simulink model "DSO4kW"  (R2024a)
settings: Solver=ode23tb  StartTime=0.0  StopTime=1  MaxStep=1e-5  RelTol=1e-6  AbsTol=1e-6
libraries: spsDiodeLib x10, spsPVArrayLib x9, spsSeriesRLCBranchLib x4, spsCurrentMeasurementLib x2, spsFirstOrderFilterLib x2, spsVoltageMeasurementLib x2, spsIGBTDiodeLib x1, spsPWMGeneratorDCDCLib x1, sps_lib x1
settings Model: Creator=Rahuldev  LastModifiedBy=Rahuldev

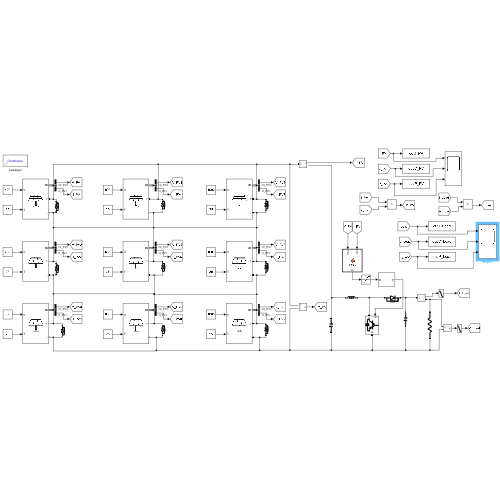
[thumbnail: Simulink's stored preview of the top-level diagram]
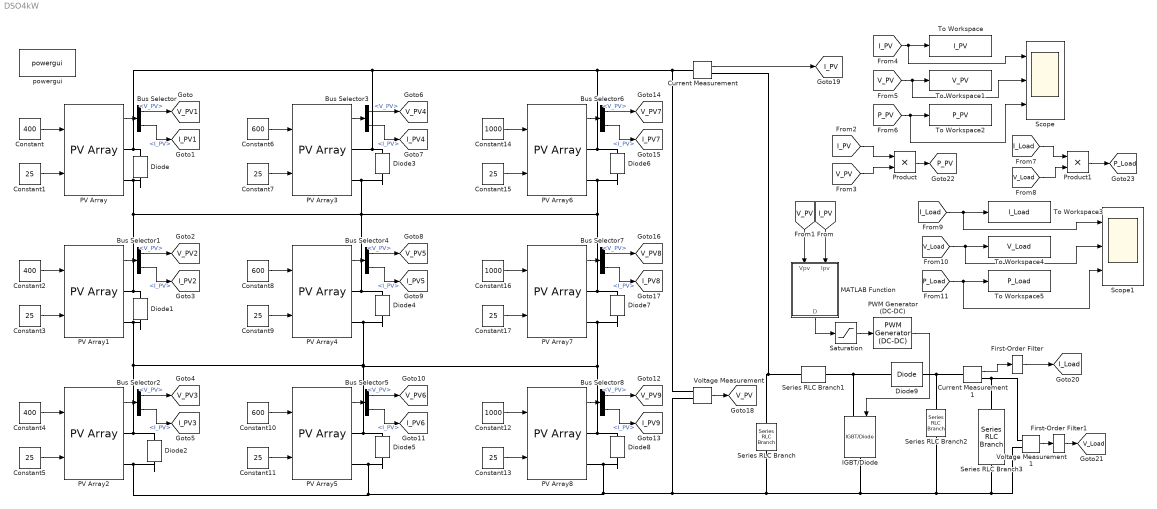
== system DSO4kW ==
  Bus Selector{,1..8} (9 alike) : BusSelector  OutputSignals=V_PV,I_PV
  Constant : Constant  Value=400
  Constant{1,3,5,7,9,11,13,15,17} (9 alike) : Constant  Value=25
  Constant10 : Constant  Value=600
  Constant12 : Constant  Value=1000
  Constant14 : Constant  Value=1000
  Constant16 : Constant  Value=1000
  Constant2 : Constant  Value=400
  Constant4 : Constant  Value=400
  Constant6 : Constant  Value=600
  Constant8 : Constant  Value=600
  Current Measurement : spsCurrentMeasurementLib/Current Measurement  PhasorSimulation=off  OutputType=Complex  PSBequivalent=0
  Current Measurement1 : spsCurrentMeasurementLib/Current Measurement  PhasorSimulation=off  OutputType=Complex  PSBequivalent=0
  Diode{,1..9} (10 alike) : spsDiodeLib/Diode  Ron=0.001  Lon=0  Vf=0.8  IC=0  UseSnubber=0  Rs=500  Cs=250e-9  Measurements=off
  First-Order Filter : spsFirstOrderFilterLib/First-Order Filter  FilterType=Lowpass  Tc=10e-3  Ts=0  Initialize=off  Vac_Init=[0, 0, 60]  Vdc_Init=0  PlotResponse=off  FreqRange="[0,  200,  1]"
  First-Order Filter1 : spsFirstOrderFilterLib/First-Order Filter  FilterType=Lowpass  Tc=10e-3  Ts=0  Initialize=off  Vac_Init=[0, 0, 60]  Vdc_Init=0  PlotResponse=off  FreqRange="[0,  200,  1]"
  IGBT/Diode : spsIGBTDiodeLib/IGBT//Diode  Ron=1e-3  Rs=1e5  Cs=inf  Measurements=off
  MATLAB Function : MATLAB Function  TreatAsAtomicUnit=on
  PV Array{,1..8} (9 alike) : spsPVArrayLib/PV Array  Npar=1  Nser=1  PlotType=array @ 25 deg.C & specified irradiances  S_vec="[ 1000  800  600  400  200 ]"  Temp_C_vec="[ 45 25  ]"  ModuleName=User-defined  PlotWhenSelected=off  Pm=540.474  Ncell=144  Voc=49.32  Isc=13.71  Vm=41.80  Im=12.93  beta_Voc_pc=-0.28  alpha_Isc_pc=0.048  beta_Voc=-0.1381  alpha_Isc=0.0065808  IL=13.7275  I0=1.9489e-11  nI=0.48903  Rsh=175.1393  Rs=0.14047  RobustModel=off  RobustCellTemperature=313.3991  BAL=on  Tc=1e-6  Tfilter=5e-5
  PWM Generator (DC-DC) : spsPWMGeneratorDCDCLib/PWM Generator (DC-DC)  Fsw=50000  Ts=0
  Product : Product
  Product1 : Product
  Saturation : Saturate
  Scope : Scope  NumInputPorts=3
  Scope1 : Scope  NumInputPorts=3
  Series RLC Branch : spsSeriesRLCBranchLib/Series RLC Branch  LConnTagsString=__new0  RConnTagsString=__new0  BranchType=C  Resistance=1  Inductance=1e-3  SetiL0=off  InitialCurrent=0  Capacitance=6.274e-4  Setx0=on  InitialVoltage=0  Measurements=None
  Series RLC Branch1 : spsSeriesRLCBranchLib/Series RLC Branch  LConnTagsString=__new0  RConnTagsString=__new0  BranchType=L  Resistance=1  Inductance=2.187e-4  SetiL0=off  InitialCurrent=0  Capacitance=1e-6  Setx0=off  InitialVoltage=0  Measurements=None
  Series RLC Branch2 : spsSeriesRLCBranchLib/Series RLC Branch  LConnTagsString=__new0  RConnTagsString=__new0  BranchType=C  Resistance=1  Inductance=1e-3  SetiL0=off  InitialCurrent=0  Capacitance=3.084e-4  Setx0=on  InitialVoltage=0  Measurements=None
  Series RLC Branch3 : spsSeriesRLCBranchLib/Series RLC Branch  LConnTagsString=__new0  RConnTagsString=__new0  BranchType=R  Resistance=4.80  Inductance=1e-3  SetiL0=off  InitialCurrent=0  Capacitance=1e-6  Setx0=off  InitialVoltage=0  Measurements=None
  To Workspace : ToWorkspace  VariableName=I_PV  SaveFormat=Structure With Time  SampleTime=-1
  To Workspace1 : ToWorkspace  VariableName=V_PV  SaveFormat=Structure With Time  SampleTime=-1
  To Workspace2 : ToWorkspace  VariableName=P_PV  SaveFormat=Structure With Time  SampleTime=-1
  To Workspace3 : ToWorkspace  VariableName=I_Load  SaveFormat=Structure With Time  SampleTime=-1
  To Workspace4 : ToWorkspace  VariableName=V_Load  SaveFormat=Structure With Time  SampleTime=-1
  To Workspace5 : ToWorkspace  VariableName=P_Load  SaveFormat=Structure With Time  SampleTime=-1
  Voltage Measurement : spsVoltageMeasurementLib/Voltage Measurement  PhasorSimulation=off  OutputType=Complex  PSBequivalent=0
  Voltage Measurement1 : spsVoltageMeasurementLib/Voltage Measurement  PhasorSimulation=off  OutputType=Complex  PSBequivalent=0
  powergui : sps_lib/powergui  Priority=1  SimulationMode=Continuous  SampleTime=50e-6  frequency=60  Iterations=50  frequencyindice=0  Pbase=100e6  ErrMax=1e-4  UnitsV=kV  UnitsW=MW  buscounter=0  FunctionMessages=off  echomessages=off  EnableUseOfTLC=off  CurrentSourceSwitches=off  DisableSnubberDevices=off  DisableRonSwitches=off  DisableVfSwitches=off  DisplayEquations=off  AutomaticDiscreteSolvers=off  SolverType=Tustin/Backward Euler (TBE)  Interpol=off  ExternalGateDelay=off  methode=off  Ts=100  x0status=blocks  SPID=on  SwTol=0  HookPort=off  NonlinearTolerance=1e-4  nMaxIteration=100  ContinueOnMaxIteration=off  RestoreLinks=warning  ResistiveCurrentMeasurement=off  Frange=[0:2:500]  Ylog=off  Xlog=on  ShowGrid=off  save=off  variable=ZData  structure=0  ZoomFFT=off  StartTime=0.0  cycles=1  DisplayStyle=1  fundamental=60  FreqAxis=off  MaxFrequency=1000  frequencyindicesteady=1  RmsSteady=1  display=off
  tag scope: I_Load=global, I_PV1=global, I_PV2=global, I_PV3=global, I_PV4=global, I_PV5=global, I_PV6=global, I_PV7=global, I_PV8=global, I_PV9=global, I_PV=global, P_Load=global, P_PV=global, V_Load=global, V_PV1=global, V_PV2=global, V_PV3=global, V_PV4=global, V_PV5=global, V_PV6=global, V_PV7=global, V_PV8=global, V_PV9=global, V_PV=global
  wires:
  PV Array/1 -> Bus Selector/1
  Constant/1 -> PV Array/1
  Constant1/1 -> PV Array/2
  Bus Selector/1 -> [V_PV1]  "<V_PV>"
  Bus Selector/2 -> [I_PV1]  "<I_PV>"
  Bus Selector1/2 -> [I_PV2]  "<I_PV>"
  Bus Selector1/1 -> [V_PV2]  "<V_PV>"
  Constant3/1 -> PV Array1/2
  Constant2/1 -> PV Array1/1
  PV Array1/1 -> Bus Selector1/1
  PV Array2/1 -> Bus Selector2/1
  Constant4/1 -> PV Array2/1
  Constant5/1 -> PV Array2/2
  Bus Selector2/1 -> [V_PV3]  "<V_PV>"
  Bus Selector2/2 -> [I_PV3]  "<I_PV>"
  Bus Selector5/2 -> [I_PV6]  "<I_PV>"
  Bus Selector5/1 -> [V_PV6]  "<V_PV>"
  Constant11/1 -> PV Array5/2
  Constant10/1 -> PV Array5/1
  PV Array5/1 -> Bus Selector5/1
  PV Array4/1 -> Bus Selector4/1
  Constant8/1 -> PV Array4/1
  Constant9/1 -> PV Array4/2
  Bus Selector4/1 -> [V_PV5]  "<V_PV>"
  Bus Selector4/2 -> [I_PV5]  "<I_PV>"
  Bus Selector3/2 -> [I_PV4]  "<I_PV>"
  Bus Selector3/1 -> [V_PV4]  "<V_PV>"
  Constant7/1 -> PV Array3/2
  Constant6/1 -> PV Array3/1
  PV Array3/1 -> Bus Selector3/1
  PV Array6/1 -> Bus Selector6/1
  Constant14/1 -> PV Array6/1
  Constant15/1 -> PV Array6/2
  Bus Selector6/1 -> [V_PV7]  "<V_PV>"
  Bus Selector6/2 -> [I_PV7]  "<I_PV>"
  Bus Selector7/2 -> [I_PV8]  "<I_PV>"
  Bus Selector7/1 -> [V_PV8]  "<V_PV>"
  Constant17/1 -> PV Array7/2
  Constant16/1 -> PV Array7/1
  PV Array7/1 -> Bus Selector7/1
  PV Array8/1 -> Bus Selector8/1
  Constant12/1 -> PV Array8/1
  Constant13/1 -> PV Array8/2
  Bus Selector8/1 -> [V_PV9]  "<V_PV>"
  Bus Selector8/2 -> [I_PV9]  "<I_PV>"
  [I_PV] -> MATLAB Function/2(Ipv)
  [V_PV] -> MATLAB Function/1(Vpv)
  PWM Generator (DC-DC)/1 -> IGBT/Diode/1
  Saturation/1 -> PWM Generator (DC-DC)/1
  MATLAB Function/1(D) -> Saturation/1
  Current Measurement1/1 -> First-Order Filter/1
  First-Order Filter/1 -> [I_Load]
  Voltage Measurement1/1 -> First-Order Filter1/1
  First-Order Filter1/1 -> [V_Load]
  [I_PV] -> Product/1
  [V_PV] -> Product/2
  Product/1 -> [P_PV]
  [I_PV] -> Scope/1, To Workspace/1
  [V_PV] -> Scope/2, To Workspace1/1
  [P_PV] -> Scope/3, To Workspace2/1
  [I_Load] -> Product1/1
  [V_Load] -> Product1/2
  Product1/1 -> [P_Load]
  [I_Load] -> Scope1/1, To Workspace3/1
  [V_Load] -> Scope1/2, To Workspace4/1
  [P_Load] -> Scope1/3, To Workspace5/1
  Current Measurement/1 -> [I_PV]
  Voltage Measurement/1 -> [V_PV]
  connections:
  Diode/LConn1 -- Diode1/RConn1 -- PV Array1/RConn1 -- Diode6/LConn1 -- PV Array6/RConn2 -- Diode7/RConn1 -- PV Array7/RConn1 -- Diode3/LConn1 -- PV Array3/RConn2 -- Diode4/RConn1 -- PV Array4/RConn1 -- PV Array/RConn2
  PV Array2/RConn1 -- PV Array5/RConn1 -- Diode5/RConn1 -- Diode7/LConn1 -- PV Array7/RConn2 -- Diode8/RConn1 -- PV Array8/RConn1 -- PV Array4/RConn2 -- Diode4/LConn1 -- PV Array1/RConn2 -- Diode1/LConn1 -- Diode2/RConn1
  PV Array3/RConn1 -- PV Array/RConn1 -- Diode/RConn1 -- Voltage Measurement/LConn1 -- Current Measurement/LConn1 -- Diode6/RConn1 -- PV Array6/RConn1 -- Diode3/RConn1
  Series RLC Branch1/LConn1 -- Current Measurement/RConn1 -- Series RLC Branch/LConn1
  Diode8/LConn1 -- Series RLC Branch3/RConn1 -- Voltage Measurement1/LConn2 -- Series RLC Branch2/RConn1 -- IGBT/Diode/RConn1 -- Series RLC Branch/RConn1 -- Voltage Measurement/LConn2 -- Diode5/LConn1 -- PV Array5/RConn2 -- PV Array2/RConn2 -- Diode2/LConn1 -- PV Array8/RConn2
  IGBT/Diode/LConn1 -- Series RLC Branch1/RConn1 -- Diode9/LConn1
  Diode9/RConn1 -- Current Measurement1/LConn1 -- Series RLC Branch2/LConn1
  Current Measurement1/RConn1 -- Series RLC Branch3/LConn1 -- Voltage Measurement1/LConn1

== matlab function DSO4kW/MATLAB Function ==
  settings: updateMethod=DISCRETE
  data: Vpv input; D output; Ipv input
function D = DSO(Vpv, Ipv)
    persistent u;
    persistent dcurrent;
    persistent pbest;
    persistent p;
    persistent dc;
    persistent v;
    persistent counter;
    persistent gbest;

    if isempty(counter)
        counter = 0;
    end
    if isempty(dcurrent)
        dcurrent = 0.9;
    end
    if isempty(gbest)
        gbest = 0.9;
    end
    if isempty(p)
        p = zeros(4, 1);
    end
    if isempty(v)
        v = zeros(4, 1);
    end
    if isempty(pbest)
        pbest = zeros(4, 1);
    end
    if isempty(u)
        u = 1;
    end
    if isempty(dc)
        dc = [0.1910; 0.3394; 0.4279; 0.4883];
    end

    if counter >= 1 && counter < 300
        D = dcurrent;
        counter = counter + 1;
        return;
    end

    counter = 0;

    if u >= 1 && u <= 4
        if (Vpv * Ipv) > p(u)
            p(u) = Vpv * Ipv;
            pbest(u) = dcurrent;
        end
    end

    u = u + 1;
    if u == 6
        u = 1;
    end

    if u <= 4
        D = dc(u);
        dcurrent = D;
        counter = 1;
    elseif u == 5
        [~, i] = max(p);
        gbest = pbest(i);
        D = gbest;
        dcurrent = D;
        counter = 1;

        for j = 1:4
            v(j) = updatevelocity(v(j), pbest(j), dc(j), gbest);
            dc(j) = updateduty(dc(j), v(j));
        end
    else
        D = 0.1;
    end
end

function vfinal = updatevelocity(velocity, pobest, d, gwbest)
    Trial_Position = pobest;
    LocalBestPosition = gwbest;
    mui = rand;

    opCrossOver = randi(3);
    if opCrossOver == 1
        mpo = 1 - mui;
        New_Team_Position = LocalBestPosition * mpo + Trial_Position * mui;
    elseif opCrossOver == 2
        mpo = 1 - mui;
        New_Team_Position = LocalBestPosition * mpo + Trial_Position * mui;
    else
        New_Team_Position = Trial_Position;
    end

    vfinal = New_Team_Position - d;
end

function dnew = updateduty(d, v)
    dnew = d + v;
    dnew = max(0, min(1, dnew)); % Ensure duty cycle remains within bounds
end
